simulink model "InertiaWheelPendulum"  (R2020b)
settings: Solver=VariableStepAuto  StartTime=0.0  StopTime=10.0  RelTol=1e-3
settings Model: Creator=Nathan  LastModifiedBy=Nathan

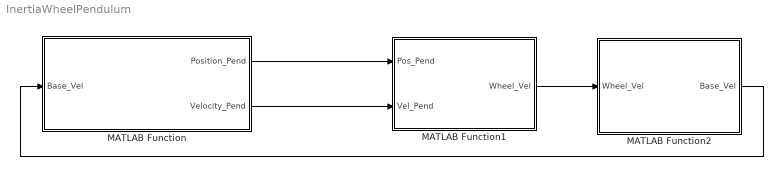
== system InertiaWheelPendulum ==
  MATLAB Function : MATLAB Function  TreatAsAtomicUnit=on
  MATLAB Function1 : MATLAB Function  TreatAsAtomicUnit=on
  MATLAB Function2 : MATLAB Function  TreatAsAtomicUnit=on
  wires:
  MATLAB Function/1(Position_Pend) -> MATLAB Function1/1(Pos_Pend)
  MATLAB Function/2(Velocity_Pend) -> MATLAB Function1/2(Vel_Pend)
  MATLAB Function1/1(Wheel_Vel) -> MATLAB Function2/1(Wheel_Vel)
  MATLAB Function2/1(Base_Vel) -> MATLAB Function/1(Base_Vel)

== matlab function InertiaWheelPendulum/MATLAB Function1 ==
  data: Pos_Pend input; Wheel_Vel output; Vel_Pend input
function Wheel_Vel = DynamicsModel(Pos_Pend,Vel_Pend)
    
    Lc1 = 2.44; %meters from base
    L1 = 2.5; %m
    m1 = 19.53; %kg
    m2 = 10; %kg
    R = 2; %m 
    
    I1 = (1/3)*m1*L1^2;
    I2 = 0.5*m2*R;
    
    K1 = 0.5*m1*Lc1^2*Vel_Pend^2 + 0.5*I1*Vel_Pend^2;
    
    syms Vel_Wheel
    
    K2 = 0.5*m2*L1^2*Vel_Pend^2 + 0.5*I2*(Vel_Pend + Vel_Wheel)^2;
    
    Vel_Sol = solve(K2 == K1, Vel_Wheel)
    
    if(Pos_Pend < 0)
        
        Wheel_Vel = Vel_Sol(1)
        
    elseif(Pos_Pend > 0)
        
        Wheel_Vel = Vel_Sol(2)
    else
        Wheel_Vel = 0;
    end
    
end

== matlab function InertiaWheelPendulum/MATLAB Function ==
  data: Position_Pend output; Velocity_Pend output; Base_Vel input
function [Position_Pend, Velocity_Pend] = SystemResponse(Base_Vel)
%      while (Base_Vel(1) > 0)
        disp('Program Started')
        sim = remApi('remoteApi');
        sim.simxFinish(-1);
        clientID = sim.simxStart('127.0.0.1',19997,true,true,5000,5);

        if(clientID > -1)
            disp('Connected to remote API Server')
            
            [res1,Base_Joint] = sim.simxGetObjectHandle(clientID,'BASE_JOINT',sim.simx_opmode_blocking);
            [res2,Wheel_Joint] = sim.simxGetObjectHandle(clientID,'WHEEL_JOINT',sim.simx_opmode_blocking);
            [res3,Pend] = sim.simxGetObjectHandle(clientID,'PENDULUM',sim.simx_opmode_blocking);
            [res4,Wheel] = sim.simxGetObjectHandle(clientID,'WHEEL',sim.simx_opmode_blocking);


            sim.simxGetObjectOrientation(clientID,Pend,-1,sim.simx_opmode_streaming);
            sim.simxGetObjectVelocity(clientID,Pend,sim.simx_opmode_streaming);
            sim.simxGetObjectVelocity(clientID,Wheel,sim.simx_opmode_streaming);

            if( res1 == sim.simx_return_ok & res2 == sim.simx_return_ok & res3 == sim.simx_return_ok & res4 == sim.simx_return_ok)
                disp('Starting Collection')
                [res] = sim.simxSetJointTargetVelocity(clientID,Base_Joint,0,sim.simx_opmode_blocking)
                
                [rtnNum, pos_pend] = sim.simxGetObjectOrientation(clientID,Pend,-1,sim.simx_opmode_buffer);
                [rtnNum2, Linvel,Angvel] = sim.simxGetObjectVelocity(clientID, Pend, sim.simx_opmode_buffer);
                [rtnNum3, Linvel_wheel,Angvel_wheel] = sim.simxGetObjectVelocity(clientID, Wheel, sim.simx_opmode_buffer);
                Position_Pend = pos_pend(1)*(180/pi)
                Velocity_Pend = Angvel(1)
                Velocity_Wheel = Angvel_wheel(3)

                sim.simxFinish(-1)
            end

        end

        sim.delete();
%      end
end

== matlab function InertiaWheelPendulum/MATLAB Function2 ==
  data: Wheel_Vel input; Base_Vel output
function Base_Vel = Controller(Wheel_Vel)
    sim = remApi('remoteApi');
    sim.simxFinish(-1);
    clientID = sim.simxStart('127.0.0.1',19997,true,true,5000,5);
    
    if(clientID > -1)
        [res,Wheel_Joint] = sim.simxGetObjectHandle(clientID,'WHEEL_JOINT',sim.simx_opmode_blocking);
        [res2,Pend] = sim.simxGetObjectHandle(clientID,'PENDULUM',sim.simx_opmode_blocking);
        sim.simxGetObjectVelocity(clientID,Pend,sim.simx_opmode_streaming);
        if(res == sim.simx_return_ok & res2 == sim.simx_return_ok)
            [Res] = sim.simxSetJointTargetVelocity(clientID,Wheel_Joint,Wheel_Vel,sim.simx_opmode_blocking)
            [Res2,Base_Vel] = sim.simxGetObjectVelocity(clientID,Pend,sim.simx_opmode_buffer)
        end
        sim.simxFinish(-1);
    end
    sim.delete();
end
